simulink model "UAV"  (R2020b)
settings: Solver=FixedStepAuto  StartTime=0.0  StopTime=20  RelTol=1e-3
values from neighbouring files (symbols this model uses):
  Body_Cd = 0.228    [Parameter.m]
  Body_G = [0,0,9.8]    [Parameter.m]
  Body_J = [Body_Jxx,0,0;0,Body_Jyy,0;0,0,Body_Jzz]    [Parameter.m]
  Body_Mass = 1.5    [Parameter.m]
  Body_R = 0.225    [Parameter.m]
  Motor_Cr = 737.24    [Parameter.m]
  Motor_Init_RPM = 557.1420    (= 557.142)    [Parameter.m]
  Motor_Jm = 2.13e-4    (= 0.000213)    [Parameter.m]
  Motor_Tm = 0.0895    [Parameter.m]
  Motor_Wb = 161.87    [Parameter.m]
  Rotor_Cm = 1.789e-7    (= 1.789e-07)    [Parameter.m]
  Rotor_Ct = 1.051e-5    (= 1.051e-05)    [Parameter.m]
libraries: sharedtransform x2, vrlib x2
settings Model: Creator=ST  LastModifiedBy=DELL
settings SolverCC: ODENIntegrationMethod=ode2
settings DebuggingCC: AlgebraicLoopMsg=none

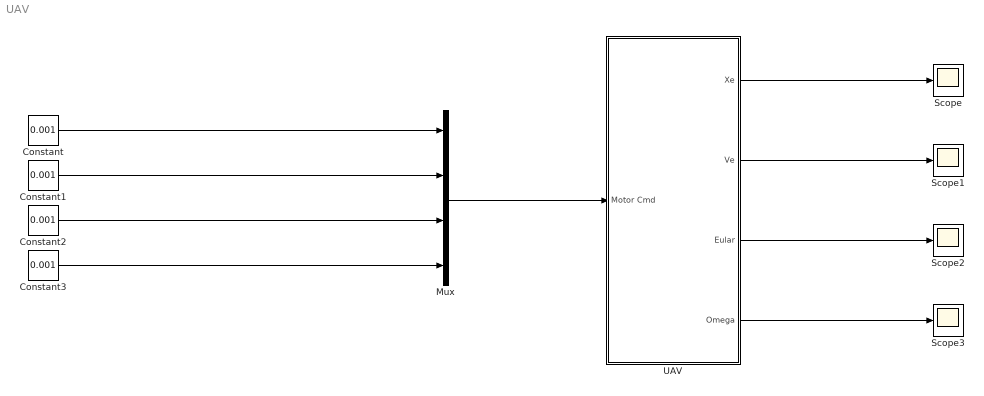
== system UAV ==
  Constant{,1..3} (4 alike) : Constant  Value=0.001
  Mux : Mux
  Scope{,1..3} (4 alike) : Scope
  UAV : Subsystem
  wires:
  UAV/4(Omega) -> Scope3/1
  UAV/3(Eular) -> Scope2/1
  UAV/2(Ve) -> Scope1/1
  UAV/1(Xe) -> Scope/1
  Mux/1 -> UAV/1(Motor Cmd)
  Constant/1 -> Mux/1
  Constant1/1 -> Mux/2
  Constant2/1 -> Mux/3
  Constant3/1 -> Mux/4

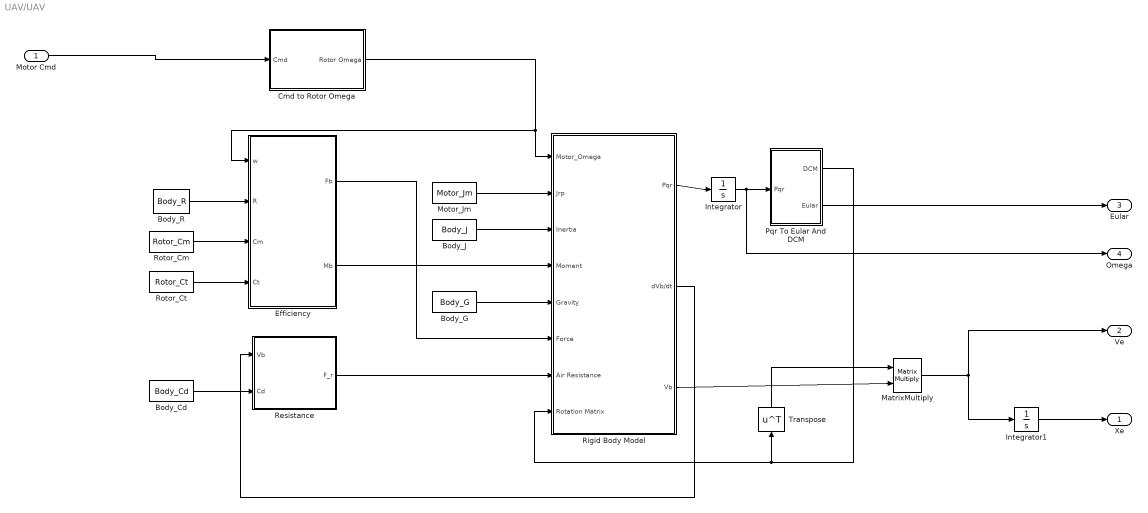
== system UAV/UAV ==
  Motor Cmd : Inport
  Body_Cd : Constant  Value=Body_Cd
  Body_G : Constant  Value=Body_G
  Body_J : Constant  Value=Body_J
  Body_R : Constant  Value=Body_R
  Cmd to Rotor Omega : Subsystem
  Efficiency : MATLAB Function  TreatAsAtomicUnit=on
  Integrator : Integrator
  Integrator1 : Integrator
  MatrixMultiply : Product  Multiplication=Matrix(*)
  Motor_Jm : Constant  Value=Motor_Jm
  Pqr To Eular And DCM : Subsystem
  Resistance : MATLAB Function  TreatAsAtomicUnit=on
  Rigid Body Model : Subsystem
  Rotor_Cm : Constant  Value=Rotor_Cm
  Rotor_Ct : Constant  Value=Rotor_Ct
  Transpose : Math  Operator=transpose  SaturateOnIntegerOverflow=on
  Xe : Outport
  Ve : Outport  Port=2
  Eular : Outport  Port=3
  Omega : Outport  Port=4
  wires:
  Efficiency/2(Mb) -> Rigid Body Model/4(Moment)
  Cmd to Rotor Omega/1(Rotor Omega) -> Efficiency/1(w), Rigid Body Model/1(Motor_Omega)
  Resistance/1(F_r) -> Rigid Body Model/7(Air Resistance)
  Integrator/1 -> Omega/1, Pqr To Eular And DCM/1(Pqr)
  Rotor_Cm/1 -> Efficiency/3(Cm)
  Efficiency/1(Fb) -> Rigid Body Model/6(Force)
  MatrixMultiply/1 -> Ve/1, Integrator1/1
  Rigid Body Model/3(Vb) -> MatrixMultiply/2
  Pqr To Eular And DCM/1(DCM) -> Transpose/1, Rigid Body Model/8(Rotation Matrix)
  Body_Cd/1 -> Resistance/2(Cd)
  Rigid Body Model/1(Pqr) -> Integrator/1
  Body_R/1 -> Efficiency/2(R)
  Body_J/1 -> Rigid Body Model/3("Inertia ")
  Rotor_Ct/1 -> Efficiency/4(Ct)
  Transpose/1 -> MatrixMultiply/1
  Rigid Body Model/2(dVb/dt) -> Resistance/1(Vb)
  Motor Cmd/1 -> Cmd to Rotor Omega/1(Cmd)
  Body_G/1 -> Rigid Body Model/5(Gravity)
  Motor_Jm/1 -> Rigid Body Model/2(Jrp)
  Pqr To Eular And DCM/2(Eular) -> Eular/1
  Integrator1/1 -> Xe/1

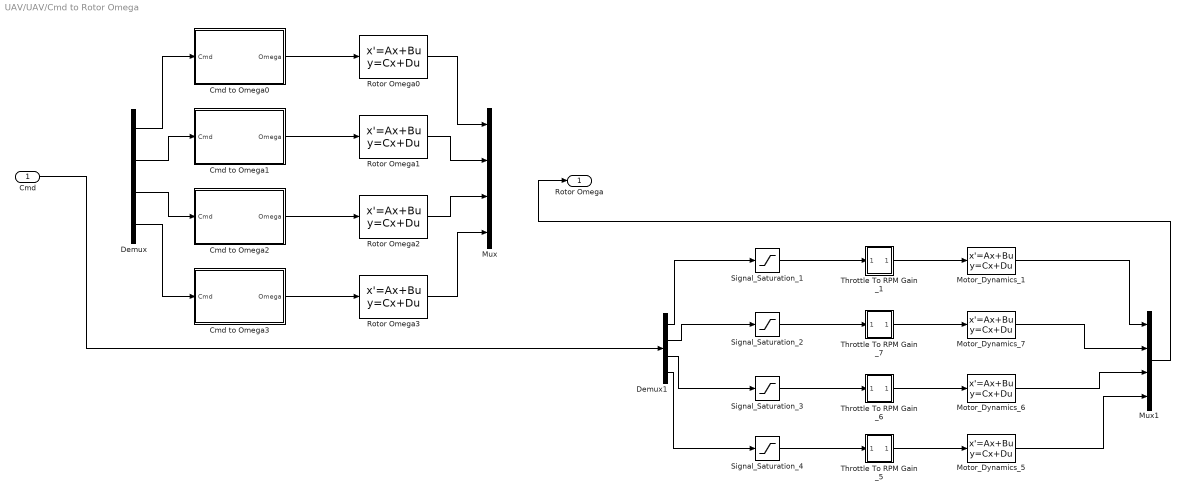
== system UAV/UAV/Cmd to Rotor Omega ==
  Cmd : Inport
  Cmd to Omega0 : Subsystem
  Cmd to Omega1 : Subsystem
  Cmd to Omega2 : Subsystem
  Cmd to Omega3 : Subsystem
  Demux : Demux
  Demux1 : Demux
  Motor_Dynamics_{1,5..7} (4 alike) : StateSpace  A=-1/Motor_Tm  C=1/Motor_Tm  D=0  InitialCondition=Motor_Init_RPM*Motor_Tm
  Mux : Mux
  Mux1 : Mux
  Rotor Omega{0..3} (4 alike) : StateSpace  A=-1/Motor_Tm  C=1/Motor_Tm  InitialCondition=0
  Signal_Saturation_{1..4} (4 alike) : Saturate  UpperLimit=1  LowerLimit=0
  Throttle To RPM Gain _1 : Subsystem
  Throttle To RPM Gain _5 : Subsystem
  Throttle To RPM Gain _6 : Subsystem
  Throttle To RPM Gain _7 : Subsystem
  Rotor Omega : Outport
  wires:
  Cmd to Omega1/1(Omega) -> Rotor Omega1/1
  Cmd to Omega2/1(Omega) -> Rotor Omega2/1
  Demux/4 -> Cmd to Omega3/1(Cmd)
  Rotor Omega3/1 -> Mux/4
  Demux/1 -> Cmd to Omega0/1(Cmd)
  Demux/2 -> Cmd to Omega1/1(Cmd)
  Cmd to Omega3/1(Omega) -> Rotor Omega3/1
  Cmd to Omega0/1(Omega) -> Rotor Omega0/1
  Demux/3 -> Cmd to Omega2/1(Cmd)
  Rotor Omega0/1 -> Mux/1
  Rotor Omega2/1 -> Mux/3
  Rotor Omega1/1 -> Mux/2
  Throttle To RPM Gain _6/1(Out5) -> Motor_Dynamics_6/1
  Throttle To RPM Gain _7/1(Out5) -> Motor_Dynamics_7/1
  Motor_Dynamics_7/1 -> Mux1/2
  Throttle To RPM Gain _5/1(Out5) -> Motor_Dynamics_5/1
  Motor_Dynamics_5/1 -> Mux1/4
  Signal_Saturation_1/1 -> Throttle To RPM Gain _1/1(In5)
  Demux1/3 -> Signal_Saturation_3/1
  Demux1/4 -> Signal_Saturation_4/1
  Throttle To RPM Gain _1/1(Out5) -> Motor_Dynamics_1/1
  Motor_Dynamics_1/1 -> Mux1/1
  Motor_Dynamics_6/1 -> Mux1/3
  Demux1/2 -> Signal_Saturation_2/1
  Demux1/1 -> Signal_Saturation_1/1
  Signal_Saturation_2/1 -> Throttle To RPM Gain _7/1(In5)
  Signal_Saturation_3/1 -> Throttle To RPM Gain _6/1(In5)
  Signal_Saturation_4/1 -> Throttle To RPM Gain _5/1(In5)
  Mux1/1 -> Rotor Omega/1
  Cmd/1 -> Demux1/1

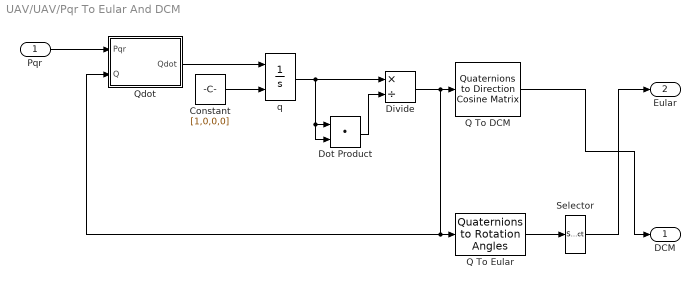
== system UAV/UAV/Pqr To Eular And DCM ==
  Pqr : Inport
  Constant : Constant  Value=[1,0,0,0]
  Divide : Product  Inputs=*/
  Dot Product : DotProduct  InputSameDT=on  OutDataTypeStr=Inherit: Inherit via internal rule
  Q To DCM : sharedtransform/Quaternions to  Direction Cosine Matrix  aMode=aMode
      settings: SourceProductBaseCode=AE,PW,MT,UV,VE,VP
  Q To Eular : sharedtransform/Quaternions to Rotation Angles  rotationOrder=ZYX  aMode=aMode
      settings: SourceProductBaseCode=AE,PW,MT,UV,VE,VP
  Qdot : MATLAB Function  TreatAsAtomicUnit=on
  Selector : Selector  InputPortWidth=3  IndexOptions=Index vector (dialog)  Indices=[3 2 1]  OutputSizes=1
  q : Integrator  InitialConditionSource=external
  DCM : Outport
  Eular : Outport  Port=2
  wires:
  Divide/1 -> Qdot/2(Q), Q To Eular/1, Q To DCM/1
  Q To DCM/1 -> DCM/1
  Q To Eular/1 -> Selector/1
  Qdot/1(Qdot) -> q/1
  q/1 -> Dot Product/2, Dot Product/1, Divide/1
  Dot Product/1 -> Divide/2
  Constant/1 -> q/2
  Pqr/1 -> Qdot/1(Pqr)
  Selector/1 -> Eular/1

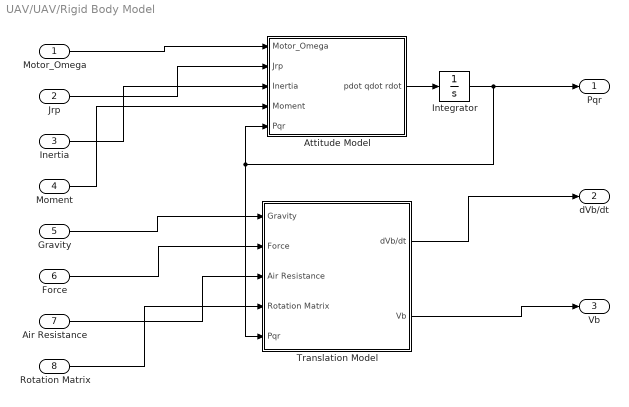
== system UAV/UAV/Rigid Body Model ==
  Motor_Omega : Inport
  Jrp : Inport  Port=2
  "Inertia " : Inport  Port=3
  Moment : Inport  Port=4
  Gravity : Inport  Port=5
  Force : Inport  Port=6
  Air Resistance : Inport  Port=7
  Rotation Matrix : Inport  Port=8
  Attitude Model : Subsystem
  Integrator : Integrator
  Translation Model : Subsystem
  Pqr : Outport
  dVb/dt : Outport  Port=2
  Vb : Outport  Port=3
  wires:
  Integrator/1 -> Pqr/1, Translation Model/5(Pqr), Attitude Model/5(Pqr)
  Gravity/1 -> Translation Model/1(Gravity)
  "Inertia "/1 -> Attitude Model/3("Inertia ")
  Attitude Model/1(pdot qdot rdot) -> Integrator/1
  Air Resistance/1 -> Translation Model/3(Air Resistance)
  Translation Model/1(dVb/dt) -> dVb/dt/1
  Jrp/1 -> Attitude Model/2(Jrp)
  Moment/1 -> Attitude Model/4(Moment)
  Rotation Matrix/1 -> Translation Model/4(Rotation Matrix)
  Translation Model/2(Vb) -> Vb/1
  Force/1 -> Translation Model/2(Force)
  Motor_Omega/1 -> Attitude Model/1(Motor_Omega)

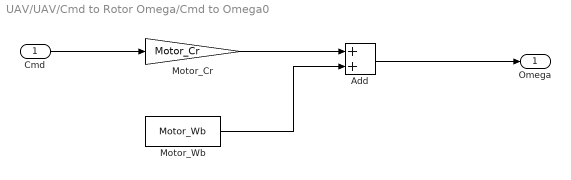
== system UAV/UAV/Cmd to Rotor Omega/Cmd to Omega0 ==
  Cmd : Inport
  Add : Sum
  Motor_Cr : Gain  Gain=Motor_Cr
  Motor_Wb : Constant  Value=Motor_Wb
  Omega : Outport
  wires:
  Cmd/1 -> Motor_Cr/1
  Motor_Cr/1 -> Add/1
  Motor_Wb/1 -> Add/2
  Add/1 -> Omega/1

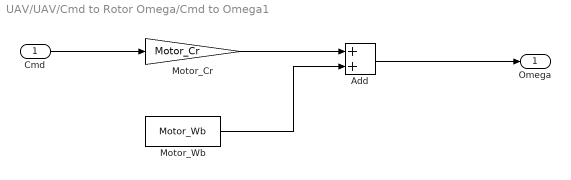
== system UAV/UAV/Cmd to Rotor Omega/Cmd to Omega1 ==
  Cmd : Inport
  Add : Sum
  Motor_Cr : Gain  Gain=Motor_Cr
  Motor_Wb : Constant  Value=Motor_Wb
  Omega : Outport
  wires:
  Cmd/1 -> Motor_Cr/1
  Motor_Cr/1 -> Add/1
  Motor_Wb/1 -> Add/2
  Add/1 -> Omega/1

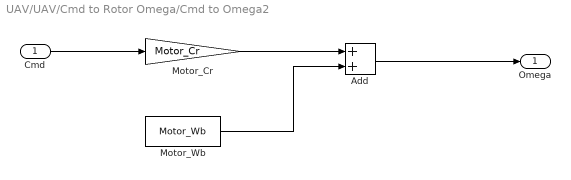
== system UAV/UAV/Cmd to Rotor Omega/Cmd to Omega2 ==
  Cmd : Inport
  Add : Sum
  Motor_Cr : Gain  Gain=Motor_Cr
  Motor_Wb : Constant  Value=Motor_Wb
  Omega : Outport
  wires:
  Cmd/1 -> Motor_Cr/1
  Motor_Cr/1 -> Add/1
  Motor_Wb/1 -> Add/2
  Add/1 -> Omega/1

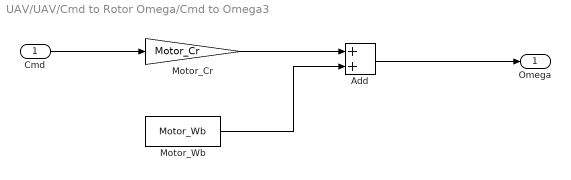
== system UAV/UAV/Cmd to Rotor Omega/Cmd to Omega3 ==
  Cmd : Inport
  Add : Sum
  Motor_Cr : Gain  Gain=Motor_Cr
  Motor_Wb : Constant  Value=Motor_Wb
  Omega : Outport
  wires:
  Cmd/1 -> Motor_Cr/1
  Motor_Cr/1 -> Add/1
  Motor_Wb/1 -> Add/2
  Add/1 -> Omega/1

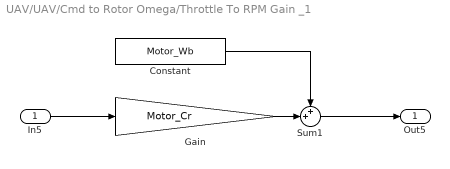
== system UAV/UAV/Cmd to Rotor Omega/Throttle To RPM Gain _1 ==
  In5 : Inport
  Constant : Constant  Value=Motor_Wb
  Gain : Gain  Gain=Motor_Cr
  Sum1 : Sum  Inputs=++|
  Out5 : Outport
  wires:
  Sum1/1 -> Out5/1
  In5/1 -> Gain/1
  Gain/1 -> Sum1/2
  Constant/1 -> Sum1/1

== system UAV/UAV/Cmd to Rotor Omega/Throttle To RPM Gain _5 ==
  In5 : Inport
  Constant : Constant  Value=Motor_Wb
  Gain : Gain  Gain=Motor_Cr
  Sum1 : Sum  Inputs=++|
  Out5 : Outport
  wires:
  Sum1/1 -> Out5/1
  In5/1 -> Gain/1
  Gain/1 -> Sum1/2
  Constant/1 -> Sum1/1

== system UAV/UAV/Cmd to Rotor Omega/Throttle To RPM Gain _6 ==
  In5 : Inport
  Constant : Constant  Value=Motor_Wb
  Gain : Gain  Gain=Motor_Cr
  Sum1 : Sum  Inputs=++|
  Out5 : Outport
  wires:
  Sum1/1 -> Out5/1
  In5/1 -> Gain/1
  Gain/1 -> Sum1/2
  Constant/1 -> Sum1/1

== system UAV/UAV/Cmd to Rotor Omega/Throttle To RPM Gain _7 ==
  In5 : Inport
  Constant : Constant  Value=Motor_Wb
  Gain : Gain  Gain=Motor_Cr
  Sum1 : Sum  Inputs=++|
  Out5 : Outport
  wires:
  Sum1/1 -> Out5/1
  In5/1 -> Gain/1
  Gain/1 -> Sum1/2
  Constant/1 -> Sum1/1

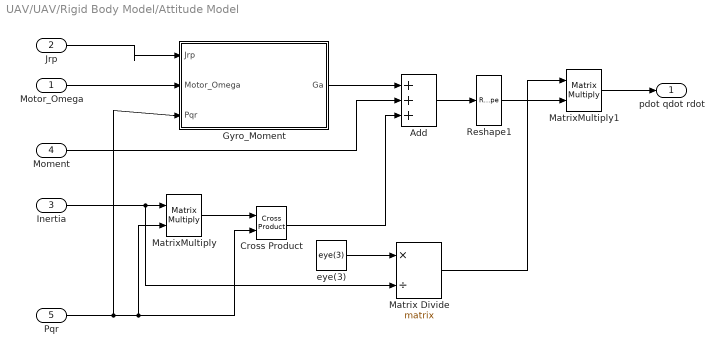
== system UAV/UAV/Rigid Body Model/Attitude Model ==
  Motor_Omega : Inport
  Jrp : Inport  Port=2
  "Inertia " : Inport  Port=3
  Moment : Inport  Port=4
  Pqr : Inport  Port=5
  Add : Sum  Inputs=+++
  Cross Product : vrlib/Utilities/Cross Product
  Gyro_Moment : MATLAB Function  TreatAsAtomicUnit=on
  Matrix Divide : Product  Inputs=*/  Multiplication=Matrix(*)
  MatrixMultiply : Product  Multiplication=Matrix(*)
  MatrixMultiply1 : Product  Multiplication=Matrix(*)
  Reshape1 : Reshape  OutputDimensionality=Column vector (2-D)
  eye(3) : Constant  Value=eye(3)
  pdot qdot rdot : Outport
  wires:
  Gyro_Moment/1(Ga) -> Add/1
  Cross Product/1 -> Add/3
  Pqr/1 -> MatrixMultiply/2, Cross Product/2, Gyro_Moment/3(Pqr)
  MatrixMultiply/1 -> Cross Product/1
  Reshape1/1 -> MatrixMultiply1/2
  Matrix Divide/1 -> MatrixMultiply1/1
  MatrixMultiply1/1 -> pdot qdot rdot/1
  "Inertia "/1 -> MatrixMultiply/1, Matrix Divide/2
  eye(3)/1 -> Matrix Divide/1
  Add/1 -> Reshape1/1
  Jrp/1 -> Gyro_Moment/1(Jrp)
  Moment/1 -> Add/2
  Motor_Omega/1 -> Gyro_Moment/2(Motor_Omega)

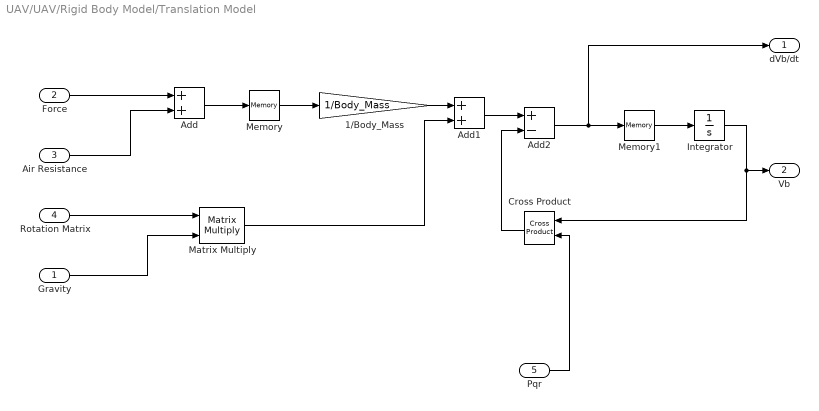
== system UAV/UAV/Rigid Body Model/Translation Model ==
  Gravity : Inport
  Force : Inport  Port=2
  Air Resistance : Inport  Port=3
  Rotation Matrix : Inport  Port=4
  Pqr : Inport  Port=5
  1/Body_Mass : Gain  Gain=1/Body_Mass
  Add : Sum
  Add1 : Sum
  Add2 : Sum  Inputs=+-
  Cross Product : vrlib/Utilities/Cross Product
  Integrator : Integrator  InitialCondition=[0,0,0]
  Matrix Multiply : Product  Multiplication=Matrix(*)
  Memory : Memory
  Memory1 : Memory
  dVb/dt : Outport
  Vb : Outport  Port=2
  wires:
  Matrix Multiply/1 -> Add1/2
  Add1/1 -> Add2/1
  Add2/1 -> Memory1/1, dVb/dt/1
  Integrator/1 -> Vb/1, Cross Product/1
  1/Body_Mass/1 -> Add1/1
  Pqr/1 -> Cross Product/2
  Force/1 -> Add/1
  Gravity/1 -> Matrix Multiply/2
  Rotation Matrix/1 -> Matrix Multiply/1
  Air Resistance/1 -> Add/2
  Memory/1 -> 1/Body_Mass/1
  Add/1 -> Memory/1
  Cross Product/1 -> Add2/2
  Memory1/1 -> Integrator/1

== matlab function UAV/Resistance ==
  data: Vb input; F_r output; Cd input
function F_r = Resistance(Vb,Cd)
F_r = Cd*Vb.*abs(Vb)*0.5;
end

== matlab function UAV/Efficiency ==
  data: w input; Fb output; R input; Cm input; Ct input; Mb output
function [Fb,Mb] = Efficiency(w,R,Cm,Ct)
%3  1
%2  4
M_Rctcm = [-sin(pi/4)*R*Ct,sin(pi/4)*R*Ct,sin(pi/4)*R*Ct,-sin(pi/4)*R*Ct;
           sin(pi/4)*R*Ct,-sin(pi/4)*R*Ct,sin(pi/4)*R*Ct,-sin(pi/4)*R*Ct;
           Cm,Cm,-Cm,-Cm];
Mb = M_Rctcm*(w.^2);
Fb = [0; 0; -sum(Ct*(w.^2))];
end

== matlab function UAV/Rigid Body Model/Attitude Model/Gyro_Moment ==
  data: Jrp input; Ga output; Motor_Omega input; Pqr input
function Ga = Gyro_Moment(Jrp,Motor_Omega,Pqr)
Ga = zeros(3,1);
Ga(1) = Jrp*Pqr(2)*(-Motor_Omega(1) - Motor_Omega(2) + Motor_Omega(3) + Motor_Omega(4));
Ga(2) = Jrp*Pqr(1)*(Motor_Omega(1) + Motor_Omega(2) - Motor_Omega(3) - Motor_Omega(4));

== matlab function UAV/Pqr To Eular And DCM/Qdot ==
  data: Pqr input; Qdot output; Q input
function Qdot = Qdot(Pqr,Q)
Qdot = 0.5 * [0,-Pqr(1),-Pqr(2),-Pqr(3);Pqr(1),0,Pqr(3),-Pqr(2);Pqr(2),-Pqr(3),0,Pqr(1);Pqr(3),Pqr(2),-Pqr(1),0] * Q;
